simulink model "MPCSmallSize"  (Simulink 8.9)
settings: Solver=ode4  StartTime=0.0  StopTime=7  FixedStep=0.001  RelTol=1e-3
InitFcn:
  | parametrosSmallSize
StopFcn:
  | robotTrajectoryAnimation(xref,yref,X(:,1),X(:,2),X(:,3))
values from neighbouring files (symbols this model uses):
  Ac = [0  wr 0 ... (first row only)    [SSmpc_ss_du_mimo.m]
  Bc = -eye(3)    [SSmpc_ss_du_mimo.m]
  C = eye(3)    [SSmpc_ss_du_mimo.m]
  T = 0.005    [SSmpc_ss_du_mimo.m]
undefined symbols (not defined in the file or in its folder): A, B
settings Model: Creator=Kawakami  LastModifiedBy=Pichau
settings DataIOCC: SignalLoggingName=sigsOut
settings OptimizationCC: BooleanDataType=off  ExpressionDepthLimit=2147483647
settings DebuggingCC: SaveWithParameterizedLinksMsg=none  SignalResolutionControl=TryResolveAllWithWarning  MultiTaskDSMMsg=warning  MultiTaskCondExecSysMsg=none
settings HardwareCC: TargetBitPerPointer=64  TargetBitPerSizeT=64  TargetBitPerPtrDiffT=64  TargetLongLongMode=on  TargetIntDivRoundTo=Zero  TargetEndianess=LittleEndian  TargetWordSize=64  TargetHWDeviceType=MATLAB Host  ProdEqTarget=off

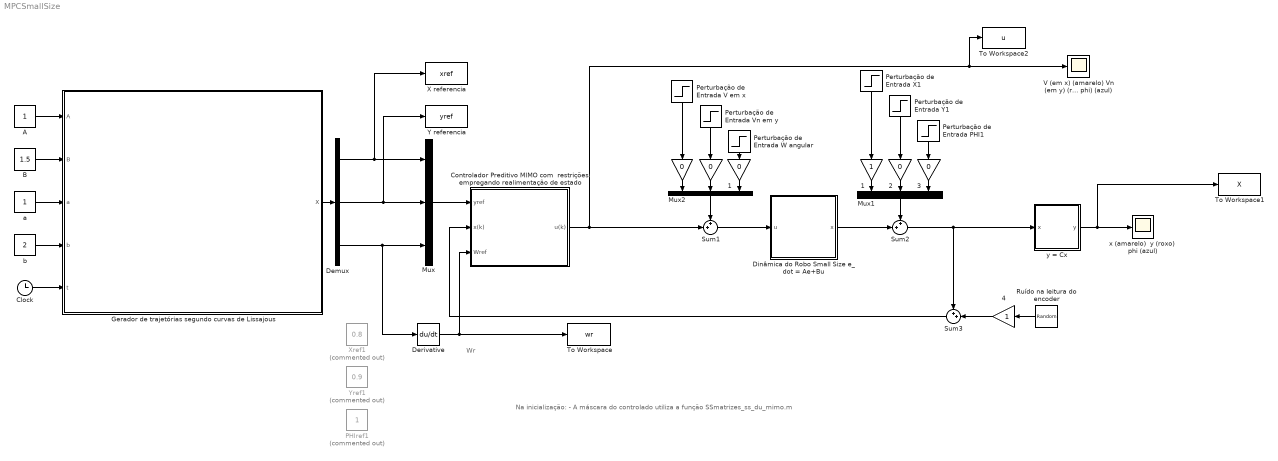
== system MPCSmallSize ==
  note: Wr
  note: Na inicialização:
      | - A máscara do controlado utiliza a função SSmatrizes_ss_du_mimo.m
   {,1..3} (4 alike) : Gain  Gain=0
  "  " : Gain  Gain=0
  "  1" : Gain
  " 4" : Gain
  " x (amarelo)  y (roxo)  phi (azul)" : Scope
  A : Constant
  B : Constant  Value=1.5
  Clock : Clock
  Controlador Preditivo MIMO com  restrições empregando realimentação de estado : Subsystem  mask{rho=[0.05;0.05;0.05], mu=[15;20;40], N=15, M=20, dulim=[-15 15;-15 15; -15 15], ulim=[-3.5 3.5;-3.5 3.5; -50 50], ylim=[-50 50;-50 50; -50 50], T=T}
      mask prompts: rho "Pesos dos controles R (p x 1)"; mu "Pesos das saídas Q (q x 1)"; N "Horizonte de Predição (N)"; M "Horizonte de Controle (M)"; dulim "[dumin,dumax] (px2)"; ulim "[umin,umax] (px2)"; ylim "[ymin,ymax] (qx2)"; T "Periodo de amostragem"
      mask init:
      | p = length(rho);
      | q = length(mu);
      | n = p;
      | umin = ulim(:,1);
      | umax = ulim(:,2);
      | dumin = dulim(:,1);
      | dumax = dulim(:,2);
      | ymin = ylim(:,1);
      | ymax = ylim(:,2);
  Demux : Demux  Outputs=3
  Derivative : Derivative
  Dinâmica do Robo Small Size e_dot = Ae+Bu : Subsystem
      mask Display: image('Glados.png');
  Gerador de trajetórias segundo curvas de Lissajous : MATLAB Function  TreatAsAtomicUnit=on
  Mux : Mux  Inputs=3
  Mux1 : Mux  Inputs=3
  Mux2 : Mux  Inputs=3
  PHIref1 : Constant  Commented=on
  Perturbação de Entrada PHI1 : Step  Time=4  After=2  SampleTime=0
  Perturbação de Entrada V em x : Step  SampleTime=0
  Perturbação de Entrada Vn em y : Step  Time=4  After=2  SampleTime=0
  Perturbação de Entrada W angular : Step  Time=4  After=2  SampleTime=0
  Perturbação de Entrada X1 : Step  Time=0.3  SampleTime=0
  Perturbação de Entrada Y1 : Step  Time=0.6  After=1.5  SampleTime=0
  Ruído na leitura do encoder : RandomNumber  Variance=0.001  SampleTime=0.1
  Sum1 : Sum  Inputs=++|  SaturateOnIntegerOverflow=on
  Sum2 : Sum  Inputs=++|  SaturateOnIntegerOverflow=on
  Sum3 : Sum  Inputs=++|  SaturateOnIntegerOverflow=on
  To Workspace : ToWorkspace  VariableName=wr  SaveFormat=Timeseries  SampleTime=-1
  To Workspace1 : ToWorkspace  VariableName=X  SampleTime=-1
      settings: Save2DSignal=2-D array (concatenate along first dimension)
  To Workspace2 : ToWorkspace  VariableName=u  SaveFormat=Structure With Time  SampleTime=-1
      settings: Save2DSignal=2-D array (concatenate along first dimension)
  V (em x) (amarelo) Vn (em y) (roxo) W (em phi) (azul) : Scope
  X referencia : ToWorkspace  VariableName=xref  SampleTime=-1
      settings: Save2DSignal=2-D array (concatenate along first dimension)
  Xref1 : Constant  Commented=on  Value=0.8
  Y referencia : ToWorkspace  VariableName=yref  SampleTime=-1
      settings: Save2DSignal=2-D array (concatenate along first dimension)
  Yref1 : Constant  Commented=on  Value=0.9
  a : Constant
  b : Constant  Value=2
  y = Cx : Subsystem
  wires:
  Controlador Preditivo MIMO com  restrições empregando realimentação de estado/1(u(k)) -> Sum1/2, To Workspace2/1, V (em x) (amarelo) Vn (em y) (roxo) W (em phi) (azul)/1
  Mux/1 -> Controlador Preditivo MIMO com  restrições empregando realimentação de estado/1(yref)
  Demux/1 -> X referencia/1, Mux/1
  Demux/2 -> Y referencia/1, Mux/2
  Sum1/1 -> Dinâmica do Robo Small Size e_dot = Ae+Bu/1(u)
  Perturbação de Entrada V em x/1 -> "  "/1
  Perturbação de Entrada Vn em y/1 -> " "/1
  "  "/1 -> Mux2/1
  " "/1 -> Mux2/2
  Derivative/1 -> Controlador Preditivo MIMO com  restrições empregando realimentação de estado/3(Wref), To Workspace/1
  Mux2/1 -> Sum1/1
  Perturbação de Entrada W angular/1 -> " 1"/1
  " 1"/1 -> Mux2/3
  y = Cx/1(y) -> To Workspace1/1, " x (amarelo)  y (roxo)  phi (azul)"/1
  Demux/3 -> Derivative/1, Mux/3
  "  1"/1 -> Mux1/1
  " 2"/1 -> Mux1/2
  Mux1/1 -> Sum2/1
  Perturbação de Entrada X1/1 -> "  1"/1
  Perturbação de Entrada Y1/1 -> " 2"/1
  Dinâmica do Robo Small Size e_dot = Ae+Bu/1(x) -> Sum2/2
  Sum2/1 -> Sum3/1, y = Cx/1(x)
  Perturbação de Entrada PHI1/1 -> " 3"/1
  " 3"/1 -> Mux1/3
  Sum3/1 -> Controlador Preditivo MIMO com  restrições empregando realimentação de estado/2(x(k))
  Ruído na leitura do encoder/1 -> " 4"/1
  " 4"/1 -> Sum3/2
  Gerador de trajetórias segundo curvas de Lissajous/1(X) -> Demux/1
  Clock/1 -> Gerador de trajetórias segundo curvas de Lissajous/5(t)
  A/1 -> Gerador de trajetórias segundo curvas de Lissajous/1(A)
  B/1 -> Gerador de trajetórias segundo curvas de Lissajous/2(B)
  a/1 -> Gerador de trajetórias segundo curvas de Lissajous/3(a)
  b/1 -> Gerador de trajetórias segundo curvas de Lissajous/4(b)

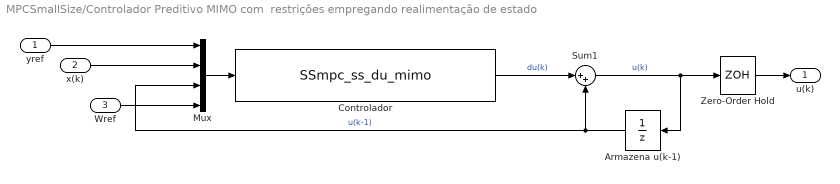
== system MPCSmallSize/Controlador Preditivo MIMO com  restrições empregando realimentação de estado ==
  yref : Inport
  x(k) : Inport  Port=2
  Wref : Inport  Port=3
  Armazena u(k-1) : UnitDelay  SampleTime=T
  Controlador : S-Function  FunctionName=SSmpc_ss_du_mimo  Parameters=dumax,dumin,umax,umin,ymax,ymin,p,q,n,N,M,mu,rho,T  SFunctionDeploymentMode=off  EnableBusSupport=off
  Mux : Mux
  Sum1 : Sum  Inputs=|++  SaturateOnIntegerOverflow=on  InputSameDT=on  OutDataTypeStr=Inherit: Same as first input
  Zero-Order Hold : ZeroOrderHold  SampleTime=T
  u(k) : Outport
  wires:
  Mux/1 -> Controlador/1
  Zero-Order Hold/1 -> u(k)/1
  x(k)/1 -> Mux/2
  yref/1 -> Mux/1
  Sum1/1 -> Zero-Order Hold/1, Armazena u(k-1)/1  "u(k)"
  Armazena u(k-1)/1 -> Sum1/2, Mux/3  "u(k-1)"
  Controlador/1 -> Sum1/1  "du(k)"
  Wref/1 -> Mux/4

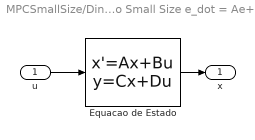
== system MPCSmallSize/Dinâmica do Robo Small Size e_dot = Ae+Bu ==
  u : Inport
  Equacao de Estado : StateSpace  A=Ac  B=Bc  C=eye(size(A,1),size(A,1))  D=zeros(size(A,1),size(B,2))  X0=zeros(size(A,1),1)
  x : Outport
  wires:
  u/1 -> Equacao de Estado/1
  Equacao de Estado/1 -> x/1

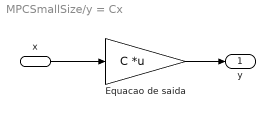
== system MPCSmallSize/y = Cx ==
  x : Inport
  Equacao de saida : Gain  Gain=C  Multiplication=Matrix(K*u)  SaturateOnIntegerOverflow=on  OutDataTypeStr=Inherit: Same as input  ParamDataTypeStr=Inherit: Same as input
  y : Outport
  wires:
  x/1 -> Equacao de saida/1
  Equacao de saida/1 -> y/1

== matlab function Gerador de trajetórias segundo curvas de Lissajous ==
  data: A input double; X output double; B input double; a input double; b input double; t input double
function X = generateLissajousTrajectory(A,B,a,b,t)

%%%%%%%%%%%%%%%%%%%%%%%%%%%%%%%%%%%%%%%%%%%%%%%%%%%%%%%%%%%%%%%%%%%%%%%%%%%
%     Função que gera os pontos de uma trajetória que segue as funções
%  de Lissajous. Feita para simulações do robô Small Size, necessita do
%  tempo de simulação e calcula o ângulo do robô com a trajetória.
%  
%     Feito em 13/05/2019
%     Autor: Arthur Azevedo
%%%%%%%%%%%%%%%%%%%%%%%%%%%%%%%%%%%%%%%%%%%%%%%%%%%%%%%%%%%%%%%%%%%%%%%%%%%

%t = linspace(0,tspan,300); %tempo total da trajetória

x = A*sin(a*t); % trajetória paramétrica em x
y = B*sin(b*t); % trajetória paramétrica em y


dx = A * a * cos(a * t); % derivada de x
dy = B * b * cos(b * t); % derivada de y

theta = atan2(dy,dx)-pi/2; % ângulo que o robô (SS) faz com a trajetória

X = [x,y,theta];
